simulink model "atthw10p5"  (R2018b)
settings: Solver=VariableStepAuto  StartTime=0.0  StopTime=6000  RelTol=1e-3
settings Model: Creator=Eric  LastModifiedBy=Eric
settings DebuggingCC: UnderSpecifiedDimensionMsg=warning

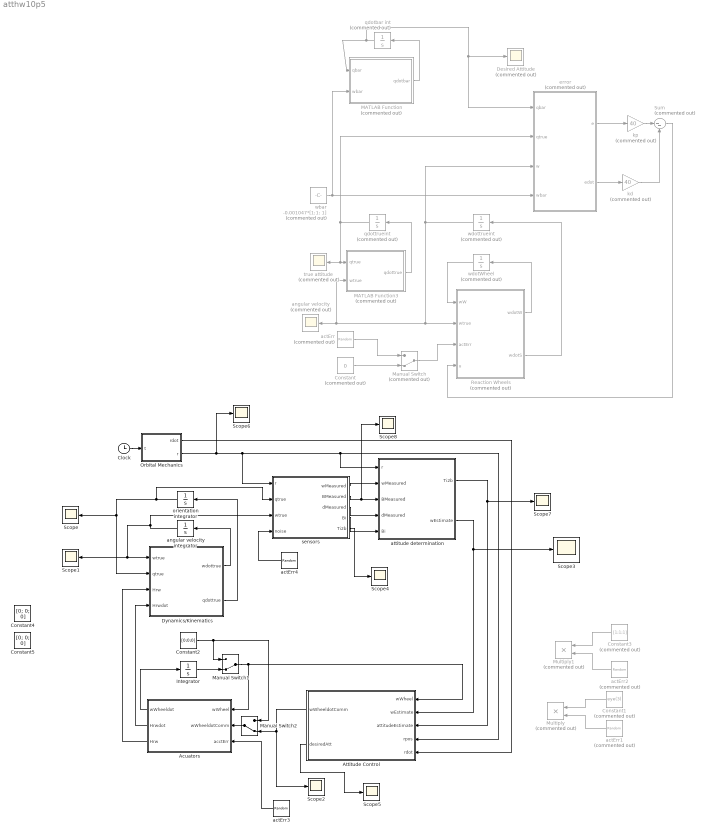
== system atthw10p5 ==
  " error " : MATLAB Function  Commented=on  TreatAsAtomicUnit=on
  Acuators : MATLAB Function  TreatAsAtomicUnit=on
  Attitude Control : MATLAB Function  TreatAsAtomicUnit=on
  Clock : Clock
  Constant : Constant  Commented=on  Value=0
  Constant1 : Constant  Commented=on  Value=eye(3)
  Constant2 : Constant  Value=[0;0;0]
  Constant3 : Constant  Commented=on  Value=[1;1;1]
  Constant4 : Constant  Value=[0; 0; 0]
  Constant5 : Constant  Value=[0; 0; 0]
  Desired Attitude : Scope  Commented=on
  Dynamics/Kinematics : MATLAB Function  TreatAsAtomicUnit=on
  Integrator : Integrator  InitialCondition=[6.92;6.92;6.92]
  MATLAB Function : MATLAB Function  Commented=on  TreatAsAtomicUnit=on
  MATLAB Function3 : MATLAB Function  Commented=on  TreatAsAtomicUnit=on
  Manual Switch : ManualSwitch  Commented=on  CurrentSetting=0
  Manual Switch1 : ManualSwitch  CurrentSetting=0
  Manual Switch2 : ManualSwitch  CurrentSetting=0
  Multiply : Product  Commented=on
  Multiply1 : Product  Commented=on
  Orbital Mechanics : MATLAB Function  TreatAsAtomicUnit=on
  "Reaction Wheels " : MATLAB Function  Commented=on  TreatAsAtomicUnit=on
  Scope{,1..8} (9 alike) : Scope
  Sum : Sum  Commented=on  Inputs=|--
  actErr : RandomNumber  Commented=on  Variance=20  SampleTime=0.1
  actErr1 : RandomNumber  Commented=on  Variance=20  SampleTime=0.1
  actErr2 : RandomNumber  Commented=on  Variance=20  SampleTime=0.1
  actErr3 : RandomNumber  Variance=20  SampleTime=0.1
  actErr4 : RandomNumber  Variance=20  SampleTime=0.1
  angular velocity : Scope  Commented=on
  angular velocity integrator : Integrator  InitialCondition=[0;0;-0.0012]
  attitude determination : MATLAB Function  TreatAsAtomicUnit=on
  kd : Gain  Commented=on  Gain=40
  kp : Gain  Commented=on  Gain=40
  orientation integrator : Integrator  InitialCondition=[0.9239;0;0.3827;0]
  qdotbar int : Integrator  Commented=on  InitialCondition=[ .5; .5; .5; .5]
  qdottrueint : Integrator  Commented=on  InitialCondition=[ .491;.491;.509;.509]/norm([ .491;.491;.509;.509])
  "sensors " : MATLAB Function  TreatAsAtomicUnit=on
  true attitude : Scope  Commented=on
  "wbar " : Constant  Commented=on  Value=-0.001047*[1;1; 1]  OutDataTypeStr=Inherit: Inherit via back propagation
  wdotWheel : Integrator  Commented=on  InitialCondition=[6.92;6.92;6.92]
  wdottrueint : Integrator  Commented=on  InitialCondition=[.01; 0; 0]
  wires:
  Sum/1 -> "Reaction Wheels "/4(u)
  actErr/1 -> Manual Switch/1
  "Reaction Wheels "/1(wdotW) -> wdotWheel/1
  MATLAB Function3/1(qdottrue) -> qdottrueint/1
  Constant/1 -> Manual Switch/2
  MATLAB Function/1(qdotbar) -> qdotbar int/1
  qdotbar int/1 -> " error "/1(qbar), Desired Attitude/1, MATLAB Function/1(qbar)
  Manual Switch/1 -> "Reaction Wheels "/3(actErr)
  kd/1 -> Sum/2
  wdotWheel/1 -> "Reaction Wheels "/1(wW)
  kp/1 -> Sum/1
  qdottrueint/1 -> " error "/2(qtrue), MATLAB Function3/1(qtrue), true attitude/1
  "wbar "/1 -> MATLAB Function/2(wbar), " error "/4(wbar)
  "Reaction Wheels "/2(wdotS) -> wdottrueint/1
  " error "/1(e) -> kp/1
  " error "/2(edot) -> kd/1
  wdottrueint/1 -> " error "/3(w), "Reaction Wheels "/2(wtrue), MATLAB Function3/2(wtrue), angular velocity/1
  Dynamics/Kinematics/1(wdottrue) -> angular velocity integrator/1
  angular velocity integrator/1 -> "sensors "/3(wtrue), Scope1/1, Dynamics/Kinematics/1(wtrue)
  Dynamics/Kinematics/2(qdottrue) -> orientation integrator/1
  orientation integrator/1 -> "sensors "/2(qtrue), Dynamics/Kinematics/2(qtrue), Scope/1
  Acuators/1(wWheeldot) -> Integrator/1
  Clock/1 -> Orbital Mechanics/1(t)
  Orbital Mechanics/1(rdot) -> Attitude Control/5(rdot)
  "sensors "/1(wMeasured) -> attitude determination/2(wMeasured)
  "sensors "/2(BMeasured) -> Scope8/1, attitude determination/3(BMeasured)
  Constant1/1 -> Multiply/1
  actErr1/1 -> Multiply/2
  Constant3/1 -> Multiply1/1
  actErr2/1 -> Multiply1/2
  actErr3/1 -> Acuators/3(acctErr)
  actErr4/1 -> "sensors "/4(noise)
  attitude determination/2(wEstimate) -> Scope3/1, Attitude Control/2(wEstimate)
  attitude determination/1(Ti2b) -> Scope7/1, Attitude Control/3(attitudeEstimate)
  "sensors "/3(dMeasured) -> attitude determination/4(dMeasured)
  Manual Switch2/1 -> Acuators/2(wWheeldotComm)
  Attitude Control/1(wWheeldotComm) -> Manual Switch2/2, Scope2/1
  "sensors "/4(Bi) -> attitude determination/5(Bi)
  "sensors "/5(Ti2b) -> Scope4/1
  Attitude Control/2(desiredAtt) -> Scope5/1
  Integrator/1 -> Manual Switch1/2
  Constant2/1 -> Manual Switch1/1, Manual Switch2/1
  Manual Switch1/1 -> Attitude Control/1(wWheel), Acuators/1(wWheel)
  Acuators/2(Hrwdot) -> Dynamics/Kinematics/4(Hrwdot)
  Acuators/3(Hrw) -> Dynamics/Kinematics/3(Hrw)
  Orbital Mechanics/2(r) -> Scope6/1, attitude determination/1(r), Attitude Control/4(rpos), "sensors "/1(r)

== matlab function atthw10p5/sensors  ==
  data: r input; qtrue input; wMeasured output; wtrue input; BMeasured output; dMeasured output; noise input; Bi output; Ti2b output
function [wMeasured, BMeasured, dMeasured, Bi, Ti2b] = sensors(r, qtrue, wtrue, noise)
noise = 0;
%
%GYRO
%

%https://www.northropgrumman.com/Capabilities/LN200FOG/Documents/ln200s.pdf
%gyro bias = 1degree/hour = 9.696E-6 rad/s
gyroBias = [0;0;0];%noise*9.696E-6*[1; 1; 1];
gyroWalk = [0;0;0];%(1/1e3)*noise*[1;1;1];
wMeasured = wtrue;% + gyroBias + gyroWalk;
qv = qtrue(2:4);
qs = qtrue(1);

skewv = [0, -qv(3), qv(2); 
         qv(3), 0, -qv(1); 
         -qv(2), qv(1), 0];
    
Ti2b = eye(3) - 2*qs*skewv + 2*skewv*skewv;

%
%MAGNETOMETER
%
magErr = [0;0;0]; %(1/1e3)*noise*[1;1;1];

Bo = 3.12E-5;
Re = 6371; %km

%DCM inertial to NEZ;
nz = -r/norm(r);
ny = (cross(nz, [0; 0; 1]))/norm(cross(nz, [0; 0; 1]));
nx = cross(ny, nz);

Ti2ned = [ nx'; ny'; nz'];


lambda = asin(r(3)/norm(r));
%magnetic field calculation
Bn = Bo*((Re/norm(r))^3)*[cos(lambda); 0; -2*sin(lambda)];
Bi = Ti2ned'*Bn; 
BMeasured = Ti2b*Bi + magErr;
BMeasured =  BMeasured/norm(BMeasured);


%
%Horizon
%
%horErr = eye(3) - (1/1e3)*noise*eye(3);
dMeasured = Ti2b*(-r/norm(r));

== matlab function atthw10p5/MATLAB Function ==
  data: qbar input; qdotbar output; wbar input
function qdotbar = qdotbar(qbar,wbar)
qwbar = .5*[0; wbar];
qdotbar = quatMult(qbar, qwbar);

== matlab function atthw10p5/ error  ==
  data: qbar input; qtrue input; e output; w input; wbar input; edot output
function [e, edot] = error(qbar, qtrue, w, wbar)
qbar(2:4) = -qbar(2:4);
dq = quatMult(qtrue, qbar);
%2
e = 2*(dq(2:4)/dq(1));

%3
dw = w - wbar;
wbskew = [0, -w(3), w(2); w(3), 0, -w(1); -w(2), w(1), 0]; 
edot = -wbskew*e + dw;

== matlab function atthw10p5/MATLAB Function3 ==
  data: qtrue input; qdottrue output; wtrue input
function qdottrue = qdottrue(qtrue, wtrue)
qwtrue = [0; wtrue];
qdottrue = .5*quatMult(qwtrue, qtrue);

== matlab function atthw10p5/Dynamics//Kinematics ==
  data: wdottrue output; wtrue input; qtrue input; Hrw input; qdottrue output; Hrwdot input
function [ wdottrue, qdottrue] = dynamics(wtrue, qtrue, Hrw, Hrwdot)
Jcg = [1000, 0, 0; 0, 500, 0; 0, 0, 600];
wdottrue = inv(Jcg)*(-cross(wtrue,Jcg*wtrue+Hrw) - Hrwdot);

qwtrue = [0; wtrue];
qdottrue = .5*quatMult(qtrue, qwtrue);

== matlab function atthw10p5/Acuators ==
  data: wWheel input; wWheeldot output; Hrwdot output; Hrw output; wWheeldotComm input; acctErr input
function [wWheeldot, Hrwdot, Hrw] = acuators( wWheel, wWheeldotComm, acctErr)
%acctErr = (.5)*rand(3,1);

wWheeldot = wWheeldotComm + acctErr*[0;0;0];

%reaction wheel specs
%http://bluecanyontech.com/rw4/
mw = 3; %kg
r = .17; %m
h = .07; %m
A = (1/12)*mw*(3*r^2 + h^2); 
C = .5*mw*r^2;

Hrwdot = C*wWheeldot;
Hrw = C*wWheel;

== matlab function atthw10p5/Reaction Wheels  ==
  data: wW input; wdotW output; wtrue input; actErr input; u input; wdotS output
function [wdotW, wdotS]    = reactionWheels(wW, wtrue, actErr, u)

%reaction wheel specs
%http://bluecanyontech.com/rw4/
mw = 3; %kg
r = .17; %m
h = .07; %m
A = (1/12)*mw*(3*r^2 + h^2); 
C = .5*mw*r^2;
Jw1 = [A, 0, 0; 0, A, 0; 0, 0, C];
Jw2 = [A, 0, 0; 0, C, 0; 0, 0, A];
Jw3 = [C, 0, 0; 0, A, 0; 0, 0, A];

% %inertia tensor of spacecraft
JcgB = [1000, 0, 0; 0, 500, 0; 0, 0, 600];
lskew = [0,-1,1;1,0,-1;-1,1,0];  %[m]. Each wheel is located along 1 meter along a body axis
JcgS = JcgB + Jw1 + Jw2 *Jw3 - 3*mw*lskew^2;
wdotW = -cross(wtrue, wW) - u - actErr;
wdotS = inv(JcgS)*(-cross(wtrue,JcgB*wtrue) - C*wdotW - cross(wtrue,C*wW));

== matlab function atthw10p5/Attitude Control ==
  data: wWheel input; wEstimate input; wWheeldotComm output; attitudeEstimate input; rpos input; rdot input; desiredAtt output
function [wWheeldotComm, desiredAtt] = attControl( wWheel, wEstimate, attitudeEstimate, rpos, rdot)
%reaction wheel specs
%http://bluecanyontech.com/rw4/
mw = 3; %kg
r = .17; %m
% h = .07; %m
% A = (1/12)*mw*(3*r^2 + h^2); 
C = .5*mw*r^2;
% Jw1 = [A, 0, 0; 0, A, 0; 0, 0, C];
% Jw2 = [A, 0, 0; 0, C, 0; 0, 0, A];
% Jw3 = [C, 0, 0; 0, A, 0; 0, 0, A];
% 
% % %inertia tensor of spacecraft
% JcgB = [1000, 0, 0; 0, 500, 0; 0, 0, 600];
% lskew = [0,-1,1;1,0,-1;-1,1,0];  %[m]. Each wheel is located along 1 meter along a body axis
JcgS = [1000, 0, 0; 0, 500, 0; 0, 0, 600];

%
%DESIRED ATTITUDE AND RATE
%
mu = 398600.4415; %km
rho = 6600; %km
w = sqrt(mu/rho^3);
wdesired = [0; 0; -w];

xbar = -rpos/norm(rpos);
zbar = cross(xbar, rdot);
zbar = zbar/norm(zbar);
ybar = cross(zbar, xbar);

desiredAtt = [xbar'; ybar'; zbar'];


%
%REACTION WHEEL COMMAND
%

attdot = attitudeEstimate*desiredAtt';
err = -.5*[attdot(3,2) - attdot(2,3); 
           attdot(1,3) - attdot(3,1); 
           attdot(2,1) - attdot(1,2)];

dw =  wEstimate - wdesired;
skewWDesired = [0,         -wdesired(3), wdesired(2);
                wdesired(3), 0,         -wdesired(1);
                -wdesired(2), wdesired(1), 0];
errdot = -skewWDesired*err + dw;
Kd = -.8;
Kp = -.8;

wWheeldotComm = -((Kp*JcgS)/C)*err - ((Kd*JcgS)/C)*errdot + cross(wEstimate, wWheel);

== matlab function atthw10p5/Orbital Mechanics ==
  data: rdot output; t input; r output
function [rdot, r] = fcn(t)
mu = 398600.4415;
rho = 6600; %km

w = sqrt(mu/rho^3);
r = (rho/sqrt(2))*[-cos(w*t); sqrt(2)*sin(w*t); cos(w*t)];
rdot = ((w*rho)/(sqrt(2)))*[sin(w*t); sqrt(2)*cos(w*t); -sin(w*t)];

== matlab function atthw10p5/attitude determination ==
  data: Ti2b output; r input; wEstimate output; wMeasured input; BMeasured input; dMeasured input; Bi input
function [Ti2b, wEstimate] = fcn(r, wMeasured, BMeasured, dMeasured, Bi)


%
%GYRO 
%

wEstimate = wMeasured;

%
%TRIAD
%


d1b = dMeasured;
d2b = BMeasured;

xb = d1b;
zb = cross(d1b, d2b)/norm(cross(d1b, d2b));
yb = cross(zb, xb);

d1i = -r/norm(r);
d2i = Bi/norm(Bi);

xi = d1i;
zi = cross(d1i, d2i)/norm(cross(d1i, d2i));
yi = cross(zi, xi);

Ti2b = [xb, yb, zb]*[xi, yi, zi]';
